simulink model "LogitechExtreme3DProRedspot"  (R2023b)
settings: Solver=VariableStepAuto  StartTime=0.0  StopTime=inf  RelTol=1e-3
undefined symbols (not defined in the file or in its folder): aircraft
libraries: vrlib x1
settings Model: Creator=jelho  LastModifiedBy=jelho

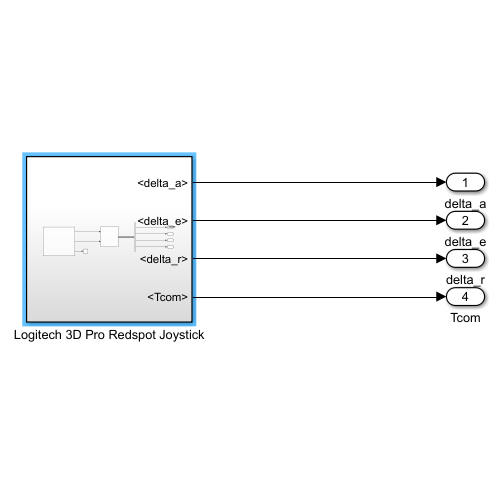
[thumbnail: Simulink's stored preview of the top-level diagram]
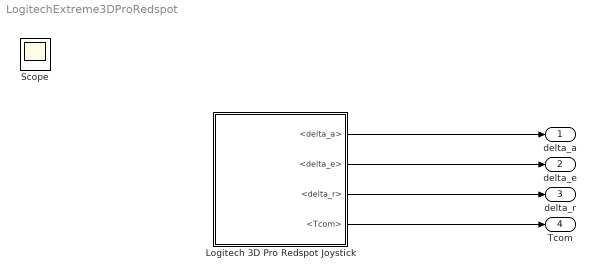
== system LogitechExtreme3DProRedspot ==
  Logitech 3D Pro Redspot Joystick : Subsystem
  delta_a : Outport
  delta_e : Outport  Port=2
  delta_r : Outport  Port=3
  Tcom : Outport  Port=4
  Scope : Scope
  wires:
  Logitech 3D Pro Redspot Joystick/1(<delta_a>) -> delta_a/1
  Logitech 3D Pro Redspot Joystick/2(<delta_e>) -> delta_e/1
  Logitech 3D Pro Redspot Joystick/3(<delta_r>) -> delta_r/1
  Logitech 3D Pro Redspot Joystick/4(<Tcom>) -> Tcom/1

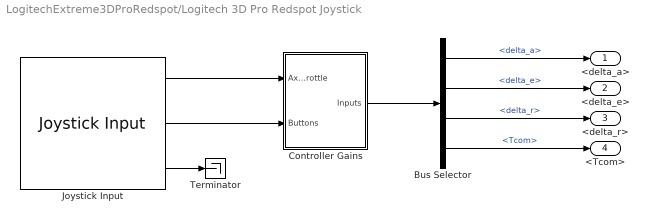
== system LogitechExtreme3DProRedspot/Logitech 3D Pro Redspot Joystick ==
  Bus Selector : BusSelector  OutputSignals=axes.delta_a,axes.delta_e,axes.delta_r,axes.Tcom
  Controller Gains : Subsystem
  Joystick Input : vrlib/Joystick Input  joyid=1  adjustports=on  forcefeed=off
  Terminator : Terminator
  <delta_a> : Outport
  <delta_e> : Outport  Port=2
  <delta_r> : Outport  Port=3
  <Tcom> : Outport  Port=4
  wires:
  Bus Selector/4 -> <Tcom>/1  "<Tcom>"
  Bus Selector/3 -> <delta_r>/1  "<delta_r>"
  Joystick Input/2 -> Controller Gains/2(Buttons)
  Joystick Input/1 -> Controller Gains/1(Axes + Throttle)
  Bus Selector/2 -> <delta_e>/1  "<delta_e>"
  Controller Gains/1(Inputs) -> Bus Selector/1
  Joystick Input/3 -> Terminator/1
  Bus Selector/1 -> <delta_a>/1  "<delta_a>"

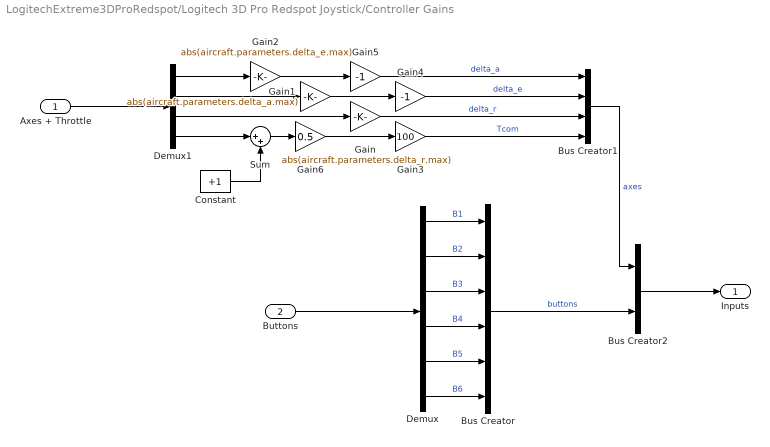
== system LogitechExtreme3DProRedspot/Logitech 3D Pro Redspot Joystick/Controller Gains ==
  Axes + Throttle : Inport
  Buttons : Inport  Port=2
  Bus Creator : BusCreator  Inputs=6
  Bus Creator1 : BusCreator  Inputs=4
  Bus Creator2 : BusCreator  Inputs=2
  Constant : Constant  Value=+1
  Demux : Demux  Outputs=6
  Demux1 : Demux
  Gain : Gain  Gain=abs(aircraft.parameters.delta_r.max)
  Gain1 : Gain  Gain=abs(aircraft.parameters.delta_a.max)
  Gain2 : Gain  Gain=abs(aircraft.parameters.delta_e.max)
  Gain3 : Gain  Gain=100
  Gain4 : Gain  Gain=-1
  Gain5 : Gain  Gain=-1
  Gain6 : Gain  Gain=0.5
  Sum : Sum  Inputs=|++
  Inputs : Outport
  wires:
  Demux1/1 -> Gain2/1
  Demux1/3 -> Gain/1
  Demux/5 -> Bus Creator/5  "B5"
  Demux1/2 -> Gain1/1
  Demux/1 -> Bus Creator/1  "B1"
  Demux/3 -> Bus Creator/3  "B3"
  Demux/2 -> Bus Creator/2  "B2"
  Demux/6 -> Bus Creator/6  "B6"
  Demux/4 -> Bus Creator/4  "B4"
  Axes + Throttle/1 -> Demux1/1
  Bus Creator1/1 -> Bus Creator2/1  "axes"
  Buttons/1 -> Demux/1
  Bus Creator/1 -> Bus Creator2/2  "buttons"
  Bus Creator2/1 -> Inputs/1
  Demux1/4 -> Sum/1
  Constant/1 -> Sum/2
  Sum/1 -> Gain6/1
  Gain/1 -> Bus Creator1/3  "delta_r"
  Gain1/1 -> Gain4/1
  Gain2/1 -> Gain5/1
  Gain3/1 -> Bus Creator1/4  "Tcom"
  Gain4/1 -> Bus Creator1/2  "delta_e"
  Gain5/1 -> Bus Creator1/1  "delta_a"
  Gain6/1 -> Gain3/1
